simulink model "MotorDiagramDerVirker"  (R2020b)
settings: Solver=VariableStepAuto  StartTime=0.0  StopTime=2  RelTol=1e-3
libraries: pid_lib x1
settings Model: Creator=henri  LastModifiedBy=henri

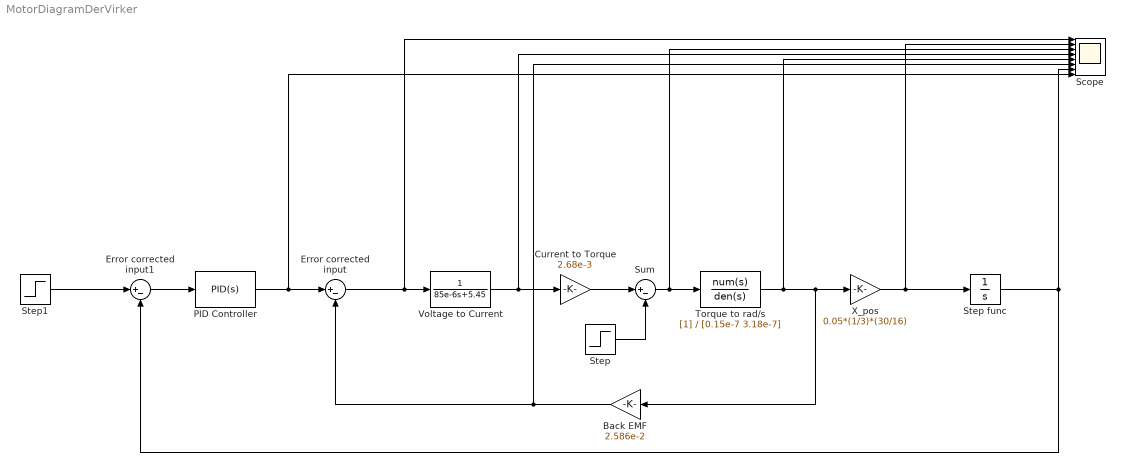
== system MotorDiagramDerVirker ==
  Back EMF : Gain  Gain=2.586e-2
  Current to Torque : Gain  Gain=2.68e-3
  Error corrected input : Sum  Inputs=|+-
  Error corrected input1 : Sum  Inputs=|+-
  PID Controller : pid_lib/PID Controller  Controller=PID  Form=Parallel  TimeDomain=Continuous-time  UseExternalTs=off  SampleTime=-1  IntegratorMethod=Forward Euler  FilterMethod=Forward Euler  ControllerParametersSource=internal  P=3342.47871920322  I=686541.066998798  D=4.05985502348164  UseFilter=on  N=475725.540003555  TunerSelectOption=Transfer Function Based (PID Tuner App)  InitialConditionSource=internal  InitialConditionForIntegrator=0  InitialConditionForFilter=0  DifferentiatorICPrevScaledInput=0  ExternalReset=none  TrackingMode=off  Kt=1  LimitOutput=on  SatLimitsSource=internal  UpperSaturationLimit=12  LowerSaturationLimit=-12  LinearizeAsGain=on  AntiWindupMode=none  Kb=1  POutMin=[]  POutMax=[]  IOutMin=[]  IOutMax=[]  DOutMin=[]  DOutMax=[]  NOutMin=[]  NOutMax=[]  SumOutMin=[]  SumOutMax=[]  SaturationOutMin=[]  SaturationOutMax=[]  PParamMin=[]  PParamMax=[]  IParamMin=[]  IParamMax=[]  DParamMin=[]  DParamMax=[]  NParamMin=[]  NParamMax=[]  KbParamMin=[]  KbParamMax=[]  KtParamMin=[]  KtParamMax=[]  KbOutMin=[]  KbOutMax=[]  KtOutMin=[]  KtOutMax=[]  IntegratorOutMin=[]  IntegratorOutMax=[]  FilterOutMin=[]  FilterOutMax=[]  SumI1OutMin=[]  SumI1OutMax=[]  SumI2OutMin=[]  SumI2OutMax=[]  SumI3OutMin=[]  SumI3OutMax=[]  SumI4OutMin=[]  SumI4OutMax=[]  SumDOutMin=[]  SumDOutMax=[]  DifferentiatorOutMin=[]  DifferentiatorOutMax=[]  FilterDiffOutCoefMin=[]  FilterDiffOutCoefMax=[]  ReciprocalOutMin=[]  ReciprocalOutMax=[]  SumDenOutMin=[]  SumDenOutMax=[]  SumNumOutMin=[]  SumNumOutMax=[]  DivideOutMin=[]  DivideOutMax=[]  UdiffTsProdOutMin=[]  UdiffTsProdOutMax=[]  NTsProdOutMin=[]  NTsProdOutMax=[]  UintegralTsProdOutMin=[]  UintegralTsProdOutMax=[]  UngainTsProdOutMin=[]  UngainTsProdOutMax=[]  IntegratorContinuousStateAttributes=''  IntegratorStateMustResolveToSignalObject=off  IntegratorRTWStateStorageClass=Auto  FilterContinuousStateAttributes=''  FilterStateMustResolveToSignalObject=off  FilterRTWStateStorageClass=Auto  ParallelPVariant=InternalParameters  IdealPVariant=Disabled  IVariant=InternalParameters  DVariant=InternalParameters  IntegratorVariant=Continuous  SatVariant=Enabled  AWVariant=Passthrough  PCopyVariant=Disabled  TRVariant=Disabled  FdbkBlocksVariant=Forward  IdealPFdbkVariant=Disabled  SatFdbkVariant=Disabled  DerivativeFilterVariant=ContFilter  NVariant=InternalParameters  NCopyVariant=Disabled  FilterICVariant=InternalICsFilter  IntegratorICVariant=InternalICs  ExternalResetVariant=Disabled  TRSumVariant=Passthrough  SumFdbkVariant=Disabled  SumVariant=Sum_PID  TsampFilterVariant=InternalTs  TsampNgainVariant=Passthrough  TsampIntegralVariant=Passthrough  ExternalSaturationOutDataTypeStr=Inherit: Same as second input
  Scope : Scope  NumInputPorts=8
  Step : Step  Time=0.8  After=1.97e-3  SampleTime=0
  Step func : Integrator
  Step1 : Step  Time=0.5  Before=0.01  After=0.1  SampleTime=0
  Sum : Sum  Inputs=|+-
  Torque to rad/s : TransferFcn  Denominator=[0.15e-7 3.18e-7]
  Voltage to Current : TransferFcn  Denominator=[85e-6 5.45]  ContinuousStateAttributes='Current'
  X_pos : Gain  Gain=0.05*(1/3)*(30/16)
  wires:
  Error corrected input/1 -> Scope/1, Voltage to Current/1
  Voltage to Current/1 -> Current to Torque/1, Scope/4
  Current to Torque/1 -> Sum/1
  Torque to rad/s/1 -> Scope/5, X_pos/1, Back EMF/1
  Back EMF/1 -> Scope/6, Error corrected input/2
  Sum/1 -> Scope/3, Torque to rad/s/1
  Step/1 -> Sum/2
  X_pos/1 -> Scope/2, Step func/1
  PID Controller/1 -> Scope/8, Error corrected input/1
  Error corrected input1/1 -> PID Controller/1
  Step1/1 -> Error corrected input1/1
  Step func/1 -> Scope/7, Error corrected input1/2
